simulink model "SIMULINK_FT_SRL_NZS_Tracking_R18b"  (R2018b)
settings: Solver=FixedStepAuto  StartTime=0.0  StopTime=sim_end_time  FixedStep=fixed_step_size  RelTol=1e-3
InitFcn:
  | start_uav_car_10
values from neighbouring files (symbols this model uses):
  a = 1    [start_uav_car_10.m]
  act_end = 2*pi/w1    (= 62.8318530718)    [start_uav_car_10.m]
  b = 1.8    [start_uav_car_10.m]
  battery_threshold = 20    [start_uav_car_10.m]
  bb = 1.2    [start_uav_car_10.m]
  delta_ = [delta_his(2:end,:); delta]    [adp_tracking.m]    (also in start_uav_car_10.m = zeros(N,1))
  draw_gif = false    [start_uav_car_10.m]
  fixed_step_size = 1/30    (= 0.0333333333333)    [start_uav_car_10.m]
  k = 0.2    [start_uav_car_10.m]
  KD_x = 0.000002    (= 2e-06)    [start_uav_car_10.m]
  KD_y = 0.00002    (= 2e-05)    [start_uav_car_10.m]
  kd_z = 0.02    [start_uav_car_10.m]
  KDD_x = 0.0008    [start_uav_car_10.m]
  KDD_y = 0.0008    [start_uav_car_10.m]
  KI_x = 0.000002    (= 2e-06)    [start_uav_car_10.m]
  KI_y = 0.000002    (= 2e-06)    [start_uav_car_10.m]
  ki_z = 0.002    [start_uav_car_10.m]
  KII_x = 0.000000    (= 0)    [start_uav_car_10.m]
  KII_y = 0.000    (= 0)    [start_uav_car_10.m]
  KP_x = 1.5    [start_uav_car_10.m]
  KP_y = 1.5    [start_uav_car_10.m]
  kp_z = 0.7    [start_uav_car_10.m]
  KPP_x = 0.4    [start_uav_car_10.m]
  KPP_y = 0.4    [start_uav_car_10.m]
  lmt = 0.5    [start_uav_car_10.m]
  omega = omega_(i,:)    [adp_tracking.m]    (also in start_uav_car_10.m = 0.3)
  omega_ = [omega_his(2:end,:); omega']    [adp_tracking.m]    (also in start_uav_car_10.m = zeros(N,l))
  R = 200*eye(2)    [adp_tracking.m]    (also in start_uav_car_10.m = 0.7)
  sim_end_time = 300    [start_uav_car_10.m]    (also in trjcar.m = 600)
  UAV_NUM = 1    [start_uav_car_10.m]
  Vel_Switch_1 = 1    [start_uav_car_10.m]
  Vel_Switch_10 = 1    [start_uav_car_10.m]
  Vel_Switch_11 = 1    [start_uav_car_10.m]
  Vel_Switch_12 = 1    [start_uav_car_10.m]
  Vel_Switch_13 = 1    [start_uav_car_10.m]
  Vel_Switch_14 = 1    [start_uav_car_10.m]
  Vel_Switch_15 = 1    [start_uav_car_10.m]
  Vel_Switch_16 = 1    [start_uav_car_10.m]
  Vel_Switch_17 = 1    [start_uav_car_10.m]
  Vel_Switch_18 = 1    [start_uav_car_10.m]
  Vel_Switch_19 = 1    [start_uav_car_10.m]
  Vel_Switch_2 = 1    [start_uav_car_10.m]
  Vel_Switch_20 = 1    [start_uav_car_10.m]
  Vel_Switch_3 = 1    [start_uav_car_10.m]
  Vel_Switch_4 = 1    [start_uav_car_10.m]
  Vel_Switch_5 = 1    [start_uav_car_10.m]
  Vel_Switch_6 = 1    [start_uav_car_10.m]
  Vel_Switch_7 = 1    [start_uav_car_10.m]
  Vel_Switch_8 = 1    [start_uav_car_10.m]
  Vel_Switch_9 = 1    [start_uav_car_10.m]
  W0 = 10*ones(l,1)    [start_uav_car_10.m]
  w1 = 0.1    [start_uav_car_10.m]
  w2 = 30    [start_uav_car_10.m]
  XMAX = 2.8    [start_uav_car_10.m]
  XMIN = -2.8    [start_uav_car_10.m]
  YMAX = 2.2    [start_uav_car_10.m]
  YMIN = -2.2    [start_uav_car_10.m]
  ys = ys_learned - ys_learned(1,:)    [start_uav_car_10.m]
  ys_learned = [-20 -19.9842645881 -19.9722755737 -19.9635643089 -19.9577075469 -19.9543235714 -19.9530686431 -19.9536337356 -19.9557415391 -19.9591437091 -19.9636183405 -19.9689676484 ... (12618 elements, 6309x2)]    [DMP_ref.mat]
  z_d_for_land = 1    [start_uav_car_10.m]
  ZMAX = 2.0    (= 2)    [start_uav_car_10.m]
  ZMIN = 0.7    [start_uav_car_10.m]
undefined symbols (not defined in the file or in its folder): droneyeeUAV2_NUM, droneyeeUAV3_NUM, droneyeeUAV4_NUM, droneyeeUAV5_NUM, uav10num, uav1num, uav2num, uav3num, uav4num, uav5num, uav6num, uav7num, uav8num, uav9num
libraries: simulink x121, aerolibanimutils x1
(part 7 of 11)

== system SIMULINK_FT_SRL_NZS_Tracking_R18b/CMD_UAV/CMD6/Subsystem ==
  clock : Inport
  uavstates : Inport  Port=2
  Constant : Constant  Value=uav6num
  MATLAB Function : MATLAB Function  TreatAsAtomicUnit=on
  "xd " : Outport
  yd : Outport  Port=2
  zd : Outport  Port=3
  wires:
  MATLAB Function/1(x_) -> "xd "/1
  MATLAB Function/2(y_) -> yd/1
  MATLAB Function/3(z_) -> zd/1
  clock/1 -> MATLAB Function/1(timestamp)
  Constant/1 -> MATLAB Function/2(uavnum)
  [switch_flag] -> MATLAB Function/3(switch_flag)
  uavstates/1 -> MATLAB Function/4(stas)
  [trj_flag] -> MATLAB Function/5(trj_flag)
  [form_flag] -> MATLAB Function/6(form_flag)
  [avo_flag] -> MATLAB Function/7(avo_flag)

== system SIMULINK_FT_SRL_NZS_Tracking_R18b/CMD_UAV/CMD7/Subsystem ==
  clock : Inport
  uavstates : Inport  Port=2
  Constant : Constant  Value=uav7num
  MATLAB Function : MATLAB Function  TreatAsAtomicUnit=on
  "xd " : Outport
  yd : Outport  Port=2
  zd : Outport  Port=3
  wires:
  uavstates/1 -> MATLAB Function/4(stas)
  [switch_flag] -> MATLAB Function/3(switch_flag)
  [avo_flag] -> MATLAB Function/7(avo_flag)
  [trj_flag] -> MATLAB Function/5(trj_flag)
  Constant/1 -> MATLAB Function/2(uavnum)
  [form_flag] -> MATLAB Function/6(form_flag)
  clock/1 -> MATLAB Function/1(timestamp)
  MATLAB Function/1(x_) -> "xd "/1
  MATLAB Function/2(y_) -> yd/1
  MATLAB Function/3(z_) -> zd/1

== system SIMULINK_FT_SRL_NZS_Tracking_R18b/CMD_UAV/CMD8/Subsystem ==
  clock : Inport
  uavstates : Inport  Port=2
  Constant : Constant  Value=uav8num
  MATLAB Function : MATLAB Function  TreatAsAtomicUnit=on
  "xd " : Outport
  yd : Outport  Port=2
  zd : Outport  Port=3
  wires:
  MATLAB Function/1(x_) -> "xd "/1
  MATLAB Function/2(y_) -> yd/1
  MATLAB Function/3(z_) -> zd/1
  clock/1 -> MATLAB Function/1(timestamp)
  Constant/1 -> MATLAB Function/2(uavnum)
  [switch_flag] -> MATLAB Function/3(switch_flag)
  uavstates/1 -> MATLAB Function/4(stas)
  [trj_flag] -> MATLAB Function/5(trj_flag)
  [form_flag] -> MATLAB Function/6(form_flag)
  [avo_flag] -> MATLAB Function/7(avo_flag)

== system SIMULINK_FT_SRL_NZS_Tracking_R18b/CMD_UAV/CMD9/Subsystem ==
  clock : Inport
  uavstates : Inport  Port=2
  Constant : Constant  Value=uav9num
  MATLAB Function : MATLAB Function  TreatAsAtomicUnit=on
  "xd " : Outport
  yd : Outport  Port=2
  zd : Outport  Port=3
  wires:
  uavstates/1 -> MATLAB Function/4(stas)
  [switch_flag] -> MATLAB Function/3(switch_flag)
  [avo_flag] -> MATLAB Function/7(avo_flag)
  [trj_flag] -> MATLAB Function/5(trj_flag)
  Constant/1 -> MATLAB Function/2(uavnum)
  [form_flag] -> MATLAB Function/6(form_flag)
  clock/1 -> MATLAB Function/1(timestamp)
  MATLAB Function/1(x_) -> "xd "/1
  MATLAB Function/2(y_) -> yd/1
  MATLAB Function/3(z_) -> zd/1

== system SIMULINK_FT_SRL_NZS_Tracking_R18b/CMD_car1/CMD1/Subsystem ==
  clock : Inport
  uavstates : Inport  Port=2
  Constant : Constant  Value=uav1num
  MATLAB Function : MATLAB Function  TreatAsAtomicUnit=on
  "xd " : Outport
  yd : Outport  Port=2
  zd : Outport  Port=3
  wires:
  MATLAB Function/1(x_) -> "xd "/1
  MATLAB Function/2(y_) -> yd/1
  MATLAB Function/3(z_) -> zd/1
  clock/1 -> MATLAB Function/1(timestamp)
  Constant/1 -> MATLAB Function/2(uavnum)
  [switch_flag] -> MATLAB Function/3(switch_flag)
  uavstates/1 -> MATLAB Function/4(stas)
  [trj_flag] -> MATLAB Function/5(trj_flag)
  [form_flag] -> MATLAB Function/6(form_flag)
  [avo_flag] -> MATLAB Function/7(avo_flag)

== system SIMULINK_FT_SRL_NZS_Tracking_R18b/CMD_car1/CMD10/Subsystem ==
  clock : Inport
  uavstates : Inport  Port=2
  Constant : Constant  Value=uav10num
  Goto : Goto  Commented=on  GotoTag=trj_flag  TagVisibility=global
  Goto1 : Goto  Commented=on  GotoTag=form_flag  TagVisibility=global
  Goto2 : Goto  Commented=on  GotoTag=avo_flag  TagVisibility=global
  MATLAB Function : MATLAB Function  TreatAsAtomicUnit=on
  轨迹 : Constant  Commented=on
  避障 : Constant  Commented=on  Value=0
  队形 : Constant  Commented=on
  "xd " : Outport
  yd : Outport  Port=2
  zd : Outport  Port=3
  wires:
  MATLAB Function/1(x_) -> "xd "/1
  MATLAB Function/2(y_) -> yd/1
  MATLAB Function/3(z_) -> zd/1
  clock/1 -> MATLAB Function/1(timestamp)
  Constant/1 -> MATLAB Function/2(uavnum)
  [switch_flag] -> MATLAB Function/3(switch_flag)
  uavstates/1 -> MATLAB Function/4(stas)
  轨迹/1 -> Goto/1
  队形/1 -> Goto1/1
  避障/1 -> Goto2/1
  [trj_flag] -> MATLAB Function/5(trj_flag)
  [form_flag] -> MATLAB Function/6(form_flag)
  [avo_flag] -> MATLAB Function/7(avo_flag)

== system SIMULINK_FT_SRL_NZS_Tracking_R18b/CMD_car1/CMD2/Subsystem ==
  clock : Inport
  uavstates : Inport  Port=2
  Constant : Constant  Value=uav2num
  MATLAB Function : MATLAB Function  TreatAsAtomicUnit=on
  "xd " : Outport
  yd : Outport  Port=2
  zd : Outport  Port=3
  wires:
  uavstates/1 -> MATLAB Function/4(stas)
  [switch_flag] -> MATLAB Function/3(switch_flag)
  [avo_flag] -> MATLAB Function/7(avo_flag)
  [trj_flag] -> MATLAB Function/5(trj_flag)
  Constant/1 -> MATLAB Function/2(uavnum)
  [form_flag] -> MATLAB Function/6(form_flag)
  clock/1 -> MATLAB Function/1(timestamp)
  MATLAB Function/1(x_) -> "xd "/1
  MATLAB Function/3(z_) -> zd/1
  MATLAB Function/2(y_) -> yd/1

== system SIMULINK_FT_SRL_NZS_Tracking_R18b/CMD_car1/CMD3/Subsystem ==
  clock : Inport
  uavstates : Inport  Port=2
  Constant : Constant  Value=uav3num
  MATLAB Function : MATLAB Function  TreatAsAtomicUnit=on
  "xd " : Outport
  yd : Outport  Port=2
  zd : Outport  Port=3
  wires:
  uavstates/1 -> MATLAB Function/4(stas)
  [switch_flag] -> MATLAB Function/3(switch_flag)
  [avo_flag] -> MATLAB Function/7(avo_flag)
  [trj_flag] -> MATLAB Function/5(trj_flag)
  Constant/1 -> MATLAB Function/2(uavnum)
  [form_flag] -> MATLAB Function/6(form_flag)
  clock/1 -> MATLAB Function/1(timestamp)
  MATLAB Function/1(x_) -> "xd "/1
  MATLAB Function/2(y_) -> yd/1
  MATLAB Function/3(z_) -> zd/1

== system SIMULINK_FT_SRL_NZS_Tracking_R18b/CMD_car1/CMD4/Subsystem ==
  clock : Inport
  uavstates : Inport  Port=2
  Constant : Constant  Value=uav4num
  MATLAB Function : MATLAB Function  TreatAsAtomicUnit=on
  "xd " : Outport
  yd : Outport  Port=2
  zd : Outport  Port=3
  wires:
  uavstates/1 -> MATLAB Function/4(stas)
  [switch_flag] -> MATLAB Function/3(switch_flag)
  [avo_flag] -> MATLAB Function/7(avo_flag)
  [trj_flag] -> MATLAB Function/5(trj_flag)
  Constant/1 -> MATLAB Function/2(uavnum)
  [form_flag] -> MATLAB Function/6(form_flag)
  clock/1 -> MATLAB Function/1(timestamp)
  MATLAB Function/1(x_) -> "xd "/1
  MATLAB Function/2(y_) -> yd/1
  MATLAB Function/3(z_) -> zd/1

== system SIMULINK_FT_SRL_NZS_Tracking_R18b/CMD_car1/CMD5/Subsystem ==
  clock : Inport
  uavstates : Inport  Port=2
  Constant : Constant  Value=uav5num
  MATLAB Function : MATLAB Function  TreatAsAtomicUnit=on
  "xd " : Outport
  yd : Outport  Port=2
  zd : Outport  Port=3
  wires:
  uavstates/1 -> MATLAB Function/4(stas)
  [switch_flag] -> MATLAB Function/3(switch_flag)
  [avo_flag] -> MATLAB Function/7(avo_flag)
  [trj_flag] -> MATLAB Function/5(trj_flag)
  Constant/1 -> MATLAB Function/2(uavnum)
  [form_flag] -> MATLAB Function/6(form_flag)
  clock/1 -> MATLAB Function/1(timestamp)
  MATLAB Function/1(x_) -> "xd "/1
  MATLAB Function/2(y_) -> yd/1
  MATLAB Function/3(z_) -> zd/1

== system SIMULINK_FT_SRL_NZS_Tracking_R18b/CMD_car1/CMD6/Subsystem ==
  clock : Inport
  uavstates : Inport  Port=2
  Constant : Constant  Value=uav6num
  MATLAB Function : MATLAB Function  TreatAsAtomicUnit=on
  "xd " : Outport
  yd : Outport  Port=2
  zd : Outport  Port=3
  wires:
  MATLAB Function/1(x_) -> "xd "/1
  MATLAB Function/2(y_) -> yd/1
  MATLAB Function/3(z_) -> zd/1
  clock/1 -> MATLAB Function/1(timestamp)
  Constant/1 -> MATLAB Function/2(uavnum)
  [switch_flag] -> MATLAB Function/3(switch_flag)
  uavstates/1 -> MATLAB Function/4(stas)
  [trj_flag] -> MATLAB Function/5(trj_flag)
  [form_flag] -> MATLAB Function/6(form_flag)
  [avo_flag] -> MATLAB Function/7(avo_flag)

== system SIMULINK_FT_SRL_NZS_Tracking_R18b/CMD_car1/CMD7/Subsystem ==
  clock : Inport
  uavstates : Inport  Port=2
  Constant : Constant  Value=uav7num
  MATLAB Function : MATLAB Function  TreatAsAtomicUnit=on
  "xd " : Outport
  yd : Outport  Port=2
  zd : Outport  Port=3
  wires:
  uavstates/1 -> MATLAB Function/4(stas)
  [switch_flag] -> MATLAB Function/3(switch_flag)
  [avo_flag] -> MATLAB Function/7(avo_flag)
  [trj_flag] -> MATLAB Function/5(trj_flag)
  Constant/1 -> MATLAB Function/2(uavnum)
  [form_flag] -> MATLAB Function/6(form_flag)
  clock/1 -> MATLAB Function/1(timestamp)
  MATLAB Function/1(x_) -> "xd "/1
  MATLAB Function/2(y_) -> yd/1
  MATLAB Function/3(z_) -> zd/1

== system SIMULINK_FT_SRL_NZS_Tracking_R18b/CMD_car1/CMD8/Subsystem ==
  clock : Inport
  uavstates : Inport  Port=2
  Constant : Constant  Value=uav8num
  MATLAB Function : MATLAB Function  TreatAsAtomicUnit=on
  "xd " : Outport
  yd : Outport  Port=2
  zd : Outport  Port=3
  wires:
  MATLAB Function/1(x_) -> "xd "/1
  MATLAB Function/2(y_) -> yd/1
  MATLAB Function/3(z_) -> zd/1
  clock/1 -> MATLAB Function/1(timestamp)
  Constant/1 -> MATLAB Function/2(uavnum)
  [switch_flag] -> MATLAB Function/3(switch_flag)
  uavstates/1 -> MATLAB Function/4(stas)
  [trj_flag] -> MATLAB Function/5(trj_flag)
  [form_flag] -> MATLAB Function/6(form_flag)
  [avo_flag] -> MATLAB Function/7(avo_flag)

== system SIMULINK_FT_SRL_NZS_Tracking_R18b/CMD_car1/CMD9/Subsystem ==
  clock : Inport
  uavstates : Inport  Port=2
  Constant : Constant  Value=uav9num
  MATLAB Function : MATLAB Function  TreatAsAtomicUnit=on
  "xd " : Outport
  yd : Outport  Port=2
  zd : Outport  Port=3
  wires:
  uavstates/1 -> MATLAB Function/4(stas)
  [switch_flag] -> MATLAB Function/3(switch_flag)
  [avo_flag] -> MATLAB Function/7(avo_flag)
  [trj_flag] -> MATLAB Function/5(trj_flag)
  Constant/1 -> MATLAB Function/2(uavnum)
  [form_flag] -> MATLAB Function/6(form_flag)
  clock/1 -> MATLAB Function/1(timestamp)
  MATLAB Function/1(x_) -> "xd "/1
  MATLAB Function/2(y_) -> yd/1
  MATLAB Function/3(z_) -> zd/1

== system SIMULINK_FT_SRL_NZS_Tracking_R18b/control system_UAV/Baseline Controller1/Heading controller ==
  yaw_e (rad) : Inport
  yaw_d. (rad) : Inport  Port=2
  Integrator Limited : Integrator  Commented=on  LimitOutput=on  UpperSaturationLimit=0.3  LowerSaturationLimit=-0.3
  Ki : Gain  Commented=on  Gain=0.01
  Sum1 : Sum  Inputs=|-+
  Sum2 : Sum  Inputs=|++
  proportional control gain - yaw : Gain  Gain=0.2
  yaw_rate_d. (rad/s) : Outport
  wires:
  Sum1/1 -> Ki/1, proportional control gain - yaw/1
  yaw_e (rad)/1 -> Sum1/1
  yaw_d. (rad)/1 -> Sum1/2
  proportional control gain - yaw/1 -> Sum2/1
  Integrator Limited/1 -> Sum2/2
  Ki/1 -> Integrator Limited/1
  Sum2/1 -> yaw_rate_d. (rad/s)/1

== system SIMULINK_FT_SRL_NZS_Tracking_R18b/control system_UAV/Baseline Controller1/Height controller  ==
  Z_d. (m) : Inport
  Z_e (m) : Inport  Port=2
  V_z : Inport  Port=3
  Discrete Derivative1 : simulink/Discrete/Discrete Derivative  gainval=1.0  ICPrevScaledInput=0.0  OutMin=[]  OutMax=[]  OutDataType=fixdt(1, 16)  OutScaling=2^-10  DoSatur=off
  Integrator Limited : Integrator  LimitOutput=on  UpperSaturationLimit=0.1  LowerSaturationLimit=-0.1
  Kd : Gain  Gain=kd_z
  Ki : Gain  Gain=ki_z
  Kp : Gain  Gain=kp_z
  Sum2 : Sum  Inputs=+++
  Sum3 : Sum  Inputs=|-+
  Z_velocity_d (m/s) : Outport
  wires:
  Sum3/1 -> Discrete Derivative1/1, Ki/1, Kp/1
  Z_e (m)/1 -> Sum3/1
  Discrete Derivative1/1 -> Kd/1
  Sum2/1 -> Z_velocity_d (m/s)/1
  Kp/1 -> Sum2/2
  Kd/1 -> Sum2/3
  Ki/1 -> Integrator Limited/1
  Integrator Limited/1 -> Sum2/1
  Z_d. (m)/1 -> Sum3/2

== system SIMULINK_FT_SRL_NZS_Tracking_R18b/control system_UAV/Baseline Controller1/Position controller ==
  X_e (m) : Inport
  Y_e (m) : Inport  Port=2
  X_d (m) : Inport  Port=3
  Y_d (m) : Inport  Port=4
  Discrete Derivative1 : simulink/Discrete/Discrete Derivative  gainval=1.0  ICPrevScaledInput=0.0  OutMin=[]  OutMax=[]  OutDataType=fixdt(1, 16)  OutScaling=2^-10  DoSatur=off
  Discrete Derivative2 : simulink/Discrete/Discrete Derivative  gainval=1.0  ICPrevScaledInput=0.0  OutMin=[]  OutMax=[]  OutDataType=fixdt(1, 16)  OutScaling=2^-10  DoSatur=off
  Integrator Limited : Integrator  LimitOutput=on  UpperSaturationLimit=0.4  LowerSaturationLimit=-0.4
  Integrator Limited1 : Integrator  LimitOutput=on  UpperSaturationLimit=0.4  LowerSaturationLimit=-0.4
  Kd : Gain  Gain=KD_x
  Kd1 : Gain  Gain=KD_y
  Kp : Gain  Gain=KP_x
  Kp1 : Gain  Gain=KI_x
  Kp2 : Gain  Gain=KP_y
  Kp3 : Gain  Gain=KI_y
  Mux : Mux  Inputs=2
  Sum2 : Sum  Inputs=+++
  Sum3 : Sum  Inputs=|-+
  Sum5 : Sum  Inputs=+++
  Sum6 : Sum  Inputs=|-+
  uxy : Outport
  wires:
  Sum5/1 -> Mux/2
  Discrete Derivative1/1 -> Kd/1
  Kp2/1 -> Sum5/2
  Sum3/1 -> Discrete Derivative1/1, Kp/1, Kp1/1
  Discrete Derivative2/1 -> Kd1/1
  X_d (m)/1 -> Sum3/2
  Integrator Limited/1 -> Sum2/1
  Y_d (m)/1 -> Sum6/2
  Kp3/1 -> Integrator Limited1/1
  Kp1/1 -> Integrator Limited/1
  Kd1/1 -> Sum5/3
  Mux/1 -> uxy/1
  Kp/1 -> Sum2/2
  X_e (m)/1 -> Sum3/1
  Integrator Limited1/1 -> Sum5/1
  Sum2/1 -> Mux/1
  Kd/1 -> Sum2/3
  Y_e (m)/1 -> Sum6/1
  Sum6/1 -> Discrete Derivative2/1, Kp2/1, Kp3/1

== system SIMULINK_FT_SRL_NZS_Tracking_R18b/control system_UAV/Baseline Controller10/Heading controller ==
  yaw_e (rad) : Inport
  yaw_d. (rad) : Inport  Port=2
  Integrator Limited : Integrator  Commented=on  LimitOutput=on  UpperSaturationLimit=0.3  LowerSaturationLimit=-0.3
  Ki : Gain  Commented=on  Gain=0.01
  Sum1 : Sum  Inputs=|-+
  Sum2 : Sum  Inputs=|++
  proportional control gain - yaw : Gain  Gain=0.2
  yaw_rate_d. (rad/s) : Outport
  wires:
  Sum1/1 -> Ki/1, proportional control gain - yaw/1
  yaw_e (rad)/1 -> Sum1/1
  yaw_d. (rad)/1 -> Sum1/2
  proportional control gain - yaw/1 -> Sum2/1
  Integrator Limited/1 -> Sum2/2
  Ki/1 -> Integrator Limited/1
  Sum2/1 -> yaw_rate_d. (rad/s)/1

== system SIMULINK_FT_SRL_NZS_Tracking_R18b/control system_UAV/Baseline Controller10/Height controller  ==
  Z_d. (m) : Inport
  Z_e (m) : Inport  Port=2
  V_z : Inport  Port=3
  Discrete Derivative1 : simulink/Discrete/Discrete Derivative  gainval=1.0  ICPrevScaledInput=0.0  OutMin=[]  OutMax=[]  OutDataType=fixdt(1, 16)  OutScaling=2^-10  DoSatur=off
  Integrator Limited : Integrator  LimitOutput=on  UpperSaturationLimit=0.1  LowerSaturationLimit=-0.1
  Kd : Gain  Gain=kd_z
  Ki : Gain  Gain=ki_z
  Kp : Gain  Gain=kp_z
  Sum2 : Sum  Inputs=+++
  Sum3 : Sum  Inputs=|-+
  Z_velocity_d (m/s) : Outport
  wires:
  Sum3/1 -> Discrete Derivative1/1, Ki/1, Kp/1
  Z_e (m)/1 -> Sum3/1
  Discrete Derivative1/1 -> Kd/1
  Sum2/1 -> Z_velocity_d (m/s)/1
  Kp/1 -> Sum2/2
  Kd/1 -> Sum2/3
  Ki/1 -> Integrator Limited/1
  Integrator Limited/1 -> Sum2/1
  Z_d. (m)/1 -> Sum3/2

== system SIMULINK_FT_SRL_NZS_Tracking_R18b/control system_UAV/Baseline Controller10/Position controller ==
  X_e (m) : Inport
  Y_e (m) : Inport  Port=2
  X_d (m) : Inport  Port=3
  Y_d (m) : Inport  Port=4
  Discrete Derivative1 : simulink/Discrete/Discrete Derivative  gainval=1.0  ICPrevScaledInput=0.0  OutMin=[]  OutMax=[]  OutDataType=fixdt(1, 16)  OutScaling=2^-10  DoSatur=off
  Discrete Derivative2 : simulink/Discrete/Discrete Derivative  gainval=1.0  ICPrevScaledInput=0.0  OutMin=[]  OutMax=[]  OutDataType=fixdt(1, 16)  OutScaling=2^-10  DoSatur=off
  Integrator Limited : Integrator  LimitOutput=on  UpperSaturationLimit=0.5  LowerSaturationLimit=-0.5
  Integrator Limited1 : Integrator  LimitOutput=on  UpperSaturationLimit=0.5  LowerSaturationLimit=-0.5
  Kd : Gain  Gain=KD_x
  Kd1 : Gain  Gain=KD_y
  Kp : Gain  Gain=KP_x
  Kp1 : Gain  Gain=KI_x
  Kp2 : Gain  Gain=KP_y
  Kp3 : Gain  Gain=KI_y
  Mux : Mux  Inputs=2
  Scope : Scope
  Scope1 : Scope
  Sum2 : Sum  Inputs=+++
  Sum3 : Sum  Inputs=|-+
  Sum5 : Sum  Inputs=+++
  Sum6 : Sum  Inputs=|-+
  uxy : Outport
  wires:
  X_e (m)/1 -> Sum3/1
  Integrator Limited/1 -> Sum2/1
  Sum2/1 -> Mux/1, Scope/1
  Kp1/1 -> Integrator Limited/1
  Kp/1 -> Sum2/2
  Kp2/1 -> Sum5/2
  Y_e (m)/1 -> Sum6/1
  Integrator Limited1/1 -> Sum5/1
  Sum5/1 -> Mux/2, Scope1/1
  Kp3/1 -> Integrator Limited1/1
  Mux/1 -> uxy/1
  X_d (m)/1 -> Sum3/2
  Discrete Derivative1/1 -> Kd/1
  Sum3/1 -> Discrete Derivative1/1, Kp/1, Kp1/1
  Y_d (m)/1 -> Sum6/2
  Sum6/1 -> Discrete Derivative2/1, Kp2/1, Kp3/1
  Kd1/1 -> Sum5/3
  Discrete Derivative2/1 -> Kd1/1
  Kd/1 -> Sum2/3

== system SIMULINK_FT_SRL_NZS_Tracking_R18b/control system_UAV/Baseline Controller2/Heading controller ==
  yaw_e (rad) : Inport
  yaw_d. (rad) : Inport  Port=2
  Integrator Limited : Integrator  Commented=on  LimitOutput=on  UpperSaturationLimit=0.3  LowerSaturationLimit=-0.3
  Ki : Gain  Commented=on  Gain=0.01
  Sum1 : Sum  Inputs=|-+
  Sum2 : Sum  Inputs=|++
  proportional control gain - yaw : Gain  Gain=0.2
  yaw_rate_d. (rad/s) : Outport
  wires:
  Sum2/1 -> yaw_rate_d. (rad/s)/1
  Ki/1 -> Integrator Limited/1
  Integrator Limited/1 -> Sum2/2
  proportional control gain - yaw/1 -> Sum2/1
  yaw_d. (rad)/1 -> Sum1/2
  yaw_e (rad)/1 -> Sum1/1
  Sum1/1 -> proportional control gain - yaw/1, Ki/1

== system SIMULINK_FT_SRL_NZS_Tracking_R18b/control system_UAV/Baseline Controller2/Height controller  ==
  Z_d. (m) : Inport
  Z_e (m) : Inport  Port=2
  V_z : Inport  Port=3
  Discrete Derivative1 : simulink/Discrete/Discrete Derivative  gainval=1.0  ICPrevScaledInput=0.0  OutMin=[]  OutMax=[]  OutDataType=fixdt(1, 16)  OutScaling=2^-10  DoSatur=off
  Integrator Limited : Integrator  LimitOutput=on  UpperSaturationLimit=0.1  LowerSaturationLimit=-0.1
  Kd : Gain  Gain=kd_z
  Ki : Gain  Gain=ki_z
  Kp : Gain  Gain=kp_z
  Sum2 : Sum  Inputs=+++
  Sum3 : Sum  Inputs=|-+
  Z_velocity_d (m/s) : Outport
  wires:
  Sum3/1 -> Discrete Derivative1/1, Ki/1, Kp/1
  Z_e (m)/1 -> Sum3/1
  Discrete Derivative1/1 -> Kd/1
  Sum2/1 -> Z_velocity_d (m/s)/1
  Kp/1 -> Sum2/2
  Kd/1 -> Sum2/3
  Ki/1 -> Integrator Limited/1
  Integrator Limited/1 -> Sum2/1
  Z_d. (m)/1 -> Sum3/2

== system SIMULINK_FT_SRL_NZS_Tracking_R18b/control system_UAV/Baseline Controller2/Position controller ==
  X_e (m) : Inport
  Y_e (m) : Inport  Port=2
  X_d (m) : Inport  Port=3
  Y_d (m) : Inport  Port=4
  Discrete Derivative1 : simulink/Discrete/Discrete Derivative  gainval=1.0  ICPrevScaledInput=0.0  OutMin=[]  OutMax=[]  OutDataType=fixdt(1, 16)  OutScaling=2^-10  DoSatur=off
  Discrete Derivative2 : simulink/Discrete/Discrete Derivative  gainval=1.0  ICPrevScaledInput=0.0  OutMin=[]  OutMax=[]  OutDataType=fixdt(1, 16)  OutScaling=2^-10  DoSatur=off
  Integrator Limited : Integrator  LimitOutput=on  UpperSaturationLimit=0.4  LowerSaturationLimit=-0.4
  Integrator Limited1 : Integrator  LimitOutput=on  UpperSaturationLimit=0.4  LowerSaturationLimit=-0.4
  Kd : Gain  Gain=KD_x
  Kd1 : Gain  Gain=KD_y
  Kp : Gain  Gain=KP_x
  Kp1 : Gain  Gain=KI_x
  Kp2 : Gain  Gain=KP_y
  Kp3 : Gain  Gain=KI_y
  Mux : Mux  Inputs=2
  Sum2 : Sum  Inputs=+++
  Sum3 : Sum  Inputs=|-+
  Sum5 : Sum  Inputs=+++
  Sum6 : Sum  Inputs=|-+
  uxy : Outport
  wires:
  Discrete Derivative2/1 -> Kd1/1
  Kd1/1 -> Sum5/3
  Sum6/1 -> Discrete Derivative2/1, Kp2/1, Kp3/1
  Y_d (m)/1 -> Sum6/2
  Kd/1 -> Sum2/3
  Discrete Derivative1/1 -> Kd/1
  Sum3/1 -> Discrete Derivative1/1, Kp1/1, Kp/1
  X_d (m)/1 -> Sum3/2
  Mux/1 -> uxy/1
  Kp3/1 -> Integrator Limited1/1
  Integrator Limited1/1 -> Sum5/1
  Y_e (m)/1 -> Sum6/1
  Kp2/1 -> Sum5/2
  Kp/1 -> Sum2/2
  Kp1/1 -> Integrator Limited/1
  Integrator Limited/1 -> Sum2/1
  X_e (m)/1 -> Sum3/1
  Sum2/1 -> Mux/1
  Sum5/1 -> Mux/2

== system SIMULINK_FT_SRL_NZS_Tracking_R18b/control system_UAV/Baseline Controller3/Heading controller ==
  yaw_e (rad) : Inport
  yaw_d. (rad) : Inport  Port=2
  Integrator Limited : Integrator  Commented=on  LimitOutput=on  UpperSaturationLimit=0.3  LowerSaturationLimit=-0.3
  Ki : Gain  Commented=on  Gain=0.01
  Sum1 : Sum  Inputs=|-+
  Sum2 : Sum  Inputs=|++
  proportional control gain - yaw : Gain  Gain=0.2
  yaw_rate_d. (rad/s) : Outport
  wires:
  Sum1/1 -> Ki/1, proportional control gain - yaw/1
  yaw_e (rad)/1 -> Sum1/1
  yaw_d. (rad)/1 -> Sum1/2
  proportional control gain - yaw/1 -> Sum2/1
  Integrator Limited/1 -> Sum2/2
  Ki/1 -> Integrator Limited/1
  Sum2/1 -> yaw_rate_d. (rad/s)/1

== system SIMULINK_FT_SRL_NZS_Tracking_R18b/control system_UAV/Baseline Controller3/Height controller  ==
  Z_d. (m) : Inport
  Z_e (m) : Inport  Port=2
  V_z : Inport  Port=3
  Discrete Derivative1 : simulink/Discrete/Discrete Derivative  gainval=1.0  ICPrevScaledInput=0.0  OutMin=[]  OutMax=[]  OutDataType=fixdt(1, 16)  OutScaling=2^-10  DoSatur=off
  Integrator Limited : Integrator  LimitOutput=on  UpperSaturationLimit=0.1  LowerSaturationLimit=-0.1
  Kd : Gain  Gain=kd_z
  Ki : Gain  Gain=ki_z
  Kp : Gain  Gain=kp_z
  Sum2 : Sum  Inputs=+++
  Sum3 : Sum  Inputs=|-+
  Z_velocity_d (m/s) : Outport
  wires:
  Sum3/1 -> Discrete Derivative1/1, Ki/1, Kp/1
  Z_e (m)/1 -> Sum3/1
  Discrete Derivative1/1 -> Kd/1
  Sum2/1 -> Z_velocity_d (m/s)/1
  Kp/1 -> Sum2/2
  Kd/1 -> Sum2/3
  Ki/1 -> Integrator Limited/1
  Integrator Limited/1 -> Sum2/1
  Z_d. (m)/1 -> Sum3/2

== system SIMULINK_FT_SRL_NZS_Tracking_R18b/control system_UAV/Baseline Controller3/Position controller ==
  X_e (m) : Inport
  Y_e (m) : Inport  Port=2
  X_d (m) : Inport  Port=3
  Y_d (m) : Inport  Port=4
  Constant : Constant  Value=0
  Discrete Derivative1 : simulink/Discrete/Discrete Derivative  gainval=1.0  ICPrevScaledInput=0.0  OutMin=[]  OutMax=[]  OutDataType=fixdt(1, 16)  OutScaling=2^-10  DoSatur=off
  Discrete Derivative2 : simulink/Discrete/Discrete Derivative  gainval=1.0  ICPrevScaledInput=0.0  OutMin=[]  OutMax=[]  OutDataType=fixdt(1, 16)  OutScaling=2^-10  DoSatur=off
  Integrator Limited : Integrator  LimitOutput=on  UpperSaturationLimit=0.5  LowerSaturationLimit=-0.5
  Integrator Limited1 : Integrator  LimitOutput=on  UpperSaturationLimit=0.5  LowerSaturationLimit=-0.5
  Kd : Gain  Gain=KD_x
  Kd1 : Gain  Gain=KD_y
  Kp : Gain  Gain=KP_x
  Kp1 : Gain  Gain=KI_x
  Kp2 : Gain  Gain=KP_y
  Kp3 : Gain  Gain=KI_y
  MATLAB Function : MATLAB Function  TreatAsAtomicUnit=on
  MATLAB Function1 : MATLAB Function  TreatAsAtomicUnit=on
  Mux : Mux  Inputs=2
  Mux1 : Mux  Inputs=2
  Mux2 : Mux  Inputs=2
  Scope1 : Scope  NumInputPorts=2
  Sum2 : Sum  Inputs=+++
  Sum3 : Sum  Inputs=|-+
  Sum5 : Sum  Inputs=+++
  Sum6 : Sum  Inputs=|-+
  Terminator : Terminator
  Terminator1 : Terminator
  To Workspace : ToWorkspace  VariableName=u  SaveFormat=Timeseries  SampleTime=-1
  To Workspace1 : ToWorkspace  VariableName=u2  SaveFormat=Timeseries  SampleTime=-1
  X-Y ADP tracking controller : Subsystem
  position_x_xd : Scope  NumInputPorts=2
  uxy : Outport
  u2xy : Outport  Port=2
  wires:
  Integrator Limited/1 -> Sum2/1
  Kp1/1 -> Integrator Limited/1
  Kp/1 -> Sum2/2
  Kp2/1 -> Sum5/2
  Integrator Limited1/1 -> Sum5/1
  Kp3/1 -> Integrator Limited1/1
  Mux/1 -> Terminator1/1
  Discrete Derivative1/1 -> Kd/1
  Kd/1 -> Sum2/3
  Sum3/1 -> Discrete Derivative1/1, Kp/1, Kp1/1
  Sum6/1 -> Discrete Derivative2/1, Kp2/1, Kp3/1
  Kd1/1 -> Sum5/3
  Discrete Derivative2/1 -> Kd1/1
  Sum2/1 -> Mux/1
  Sum5/1 -> Mux/2
  X-Y ADP tracking controller/2(uy) -> Scope1/2, Mux1/2
  X_d (m)/1 -> MATLAB Function/1(x), Sum3/2
  MATLAB Function1/1(p) -> position_x_xd/1, X-Y ADP tracking controller/1(Feedback1)
  Y_d (m)/1 -> MATLAB Function/2(y), Sum6/2
  X_e (m)/1 -> MATLAB Function1/1(x), Sum3/1
  Mux1/1 -> To Workspace/1, uxy/1
  X-Y ADP tracking controller/3(" p_virtual1") -> Terminator/1
  Y_e (m)/1 -> MATLAB Function1/2(y), Sum6/1
  MATLAB Function/1(p) -> position_x_xd/2, X-Y ADP tracking controller/3(p_virtual)
  X-Y ADP tracking controller/1(ux) -> Mux1/1, Scope1/1
  Constant/1 -> X-Y ADP tracking controller/2(Joystick)
  Mux2/1 -> u2xy/1, To Workspace1/1
  X-Y ADP tracking controller/4(u2x) -> Mux2/1
  X-Y ADP tracking controller/5(u2y) -> Mux2/2

== system SIMULINK_FT_SRL_NZS_Tracking_R18b/control system_UAV/Baseline Controller4/Heading controller ==
  yaw_e (rad) : Inport
  yaw_d. (rad) : Inport  Port=2
  Integrator Limited : Integrator  Commented=on  LimitOutput=on  UpperSaturationLimit=0.3  LowerSaturationLimit=-0.3
  Ki : Gain  Commented=on  Gain=0.01
  Sum1 : Sum  Inputs=|-+
  Sum2 : Sum  Inputs=|++
  proportional control gain - yaw : Gain  Gain=0.2
  yaw_rate_d. (rad/s) : Outport
  wires:
  Sum2/1 -> yaw_rate_d. (rad/s)/1
  Ki/1 -> Integrator Limited/1
  Integrator Limited/1 -> Sum2/2
  proportional control gain - yaw/1 -> Sum2/1
  yaw_d. (rad)/1 -> Sum1/2
  yaw_e (rad)/1 -> Sum1/1
  Sum1/1 -> proportional control gain - yaw/1, Ki/1

== system SIMULINK_FT_SRL_NZS_Tracking_R18b/control system_UAV/Baseline Controller4/Height controller  ==
  Z_d. (m) : Inport
  Z_e (m) : Inport  Port=2
  V_z : Inport  Port=3
  Discrete Derivative1 : simulink/Discrete/Discrete Derivative  gainval=1.0  ICPrevScaledInput=0.0  OutMin=[]  OutMax=[]  OutDataType=fixdt(1, 16)  OutScaling=2^-10  DoSatur=off
  Integrator Limited : Integrator  LimitOutput=on  UpperSaturationLimit=0.1  LowerSaturationLimit=-0.1
  Kd : Gain  Gain=kd_z
  Ki : Gain  Gain=ki_z
  Kp : Gain  Gain=kp_z
  Sum2 : Sum  Inputs=+++
  Sum3 : Sum  Inputs=|-+
  Z_velocity_d (m/s) : Outport
  wires:
  Sum3/1 -> Discrete Derivative1/1, Ki/1, Kp/1
  Z_e (m)/1 -> Sum3/1
  Discrete Derivative1/1 -> Kd/1
  Sum2/1 -> Z_velocity_d (m/s)/1
  Kp/1 -> Sum2/2
  Kd/1 -> Sum2/3
  Ki/1 -> Integrator Limited/1
  Integrator Limited/1 -> Sum2/1
  Z_d. (m)/1 -> Sum3/2

== system SIMULINK_FT_SRL_NZS_Tracking_R18b/control system_UAV/Baseline Controller4/Position controller ==
  X_e (m) : Inport
  Y_e (m) : Inport  Port=2
  X_d (m) : Inport  Port=3
  Y_d (m) : Inport  Port=4
  Discrete Derivative1 : simulink/Discrete/Discrete Derivative  gainval=1.0  ICPrevScaledInput=0.0  OutMin=[]  OutMax=[]  OutDataType=fixdt(1, 16)  OutScaling=2^-10  DoSatur=off
  Discrete Derivative2 : simulink/Discrete/Discrete Derivative  gainval=1.0  ICPrevScaledInput=0.0  OutMin=[]  OutMax=[]  OutDataType=fixdt(1, 16)  OutScaling=2^-10  DoSatur=off
  Integrator Limited : Integrator  LimitOutput=on  UpperSaturationLimit=0.5  LowerSaturationLimit=-0.5
  Integrator Limited1 : Integrator  LimitOutput=on  UpperSaturationLimit=0.5  LowerSaturationLimit=-0.5
  Kd : Gain  Gain=KD_x
  Kd1 : Gain  Gain=KD_y
  Kp : Gain  Gain=KP_x
  Kp1 : Gain  Gain=KI_x
  Kp2 : Gain  Gain=KP_y
  Kp3 : Gain  Gain=KI_y
  Mux : Mux  Inputs=2
  Sum2 : Sum  Inputs=+++
  Sum3 : Sum  Inputs=|-+
  Sum5 : Sum  Inputs=+++
  Sum6 : Sum  Inputs=|-+
  uxy : Outport
  wires:
  Discrete Derivative2/1 -> Kd1/1
  Kd1/1 -> Sum5/3
  Sum6/1 -> Discrete Derivative2/1, Kp3/1, Kp2/1
  Y_d (m)/1 -> Sum6/2
  Sum3/1 -> Discrete Derivative1/1, Kp1/1, Kp/1
  Kd/1 -> Sum2/3
  Discrete Derivative1/1 -> Kd/1
  X_d (m)/1 -> Sum3/2
  Mux/1 -> uxy/1
  Kp3/1 -> Integrator Limited1/1
  Integrator Limited1/1 -> Sum5/1
  Y_e (m)/1 -> Sum6/1
  Kp2/1 -> Sum5/2
  Kp/1 -> Sum2/2
  Kp1/1 -> Integrator Limited/1
  Integrator Limited/1 -> Sum2/1
  X_e (m)/1 -> Sum3/1
  Sum5/1 -> Mux/2
  Sum2/1 -> Mux/1

== system SIMULINK_FT_SRL_NZS_Tracking_R18b/control system_UAV/Baseline Controller5/Heading controller ==
  yaw_e (rad) : Inport
  yaw_d. (rad) : Inport  Port=2
  Integrator Limited : Integrator  Commented=on  LimitOutput=on  UpperSaturationLimit=0.3  LowerSaturationLimit=-0.3
  Ki : Gain  Commented=on  Gain=0.01
  Sum1 : Sum  Inputs=|-+
  Sum2 : Sum  Inputs=|++
  proportional control gain - yaw : Gain  Gain=0.2
  yaw_rate_d. (rad/s) : Outport
  wires:
  Sum1/1 -> Ki/1, proportional control gain - yaw/1
  yaw_e (rad)/1 -> Sum1/1
  yaw_d. (rad)/1 -> Sum1/2
  proportional control gain - yaw/1 -> Sum2/1
  Integrator Limited/1 -> Sum2/2
  Ki/1 -> Integrator Limited/1
  Sum2/1 -> yaw_rate_d. (rad/s)/1

== system SIMULINK_FT_SRL_NZS_Tracking_R18b/control system_UAV/Baseline Controller5/Height controller  ==
  Z_d. (m) : Inport
  Z_e (m) : Inport  Port=2
  V_z : Inport  Port=3
  Discrete Derivative1 : simulink/Discrete/Discrete Derivative  gainval=1.0  ICPrevScaledInput=0.0  OutMin=[]  OutMax=[]  OutDataType=fixdt(1, 16)  OutScaling=2^-10  DoSatur=off
  Integrator Limited : Integrator  LimitOutput=on  UpperSaturationLimit=0.1  LowerSaturationLimit=-0.1
  Kd : Gain  Gain=kd_z
  Ki : Gain  Gain=ki_z
  Kp : Gain  Gain=kp_z
  Sum2 : Sum  Inputs=+++
  Sum3 : Sum  Inputs=|-+
  Z_velocity_d (m/s) : Outport
  wires:
  Sum3/1 -> Discrete Derivative1/1, Ki/1, Kp/1
  Z_e (m)/1 -> Sum3/1
  Discrete Derivative1/1 -> Kd/1
  Sum2/1 -> Z_velocity_d (m/s)/1
  Kp/1 -> Sum2/2
  Kd/1 -> Sum2/3
  Ki/1 -> Integrator Limited/1
  Integrator Limited/1 -> Sum2/1
  Z_d. (m)/1 -> Sum3/2

== system SIMULINK_FT_SRL_NZS_Tracking_R18b/control system_UAV/Baseline Controller5/Position controller ==
  X_e (m) : Inport
  Y_e (m) : Inport  Port=2
  X_d (m) : Inport  Port=3
  Y_d (m) : Inport  Port=4
  Discrete Derivative1 : simulink/Discrete/Discrete Derivative  gainval=1.0  ICPrevScaledInput=0.0  OutMin=[]  OutMax=[]  OutDataType=fixdt(1, 16)  OutScaling=2^-10  DoSatur=off
  Discrete Derivative2 : simulink/Discrete/Discrete Derivative  gainval=1.0  ICPrevScaledInput=0.0  OutMin=[]  OutMax=[]  OutDataType=fixdt(1, 16)  OutScaling=2^-10  DoSatur=off
  Integrator Limited : Integrator  LimitOutput=on  UpperSaturationLimit=0.5  LowerSaturationLimit=-0.5
  Integrator Limited1 : Integrator  LimitOutput=on  UpperSaturationLimit=0.5  LowerSaturationLimit=-0.5
  Kd : Gain  Gain=KD_x
  Kd1 : Gain  Gain=KD_y
  Kp : Gain  Gain=KP_x
  Kp1 : Gain  Gain=KI_x
  Kp2 : Gain  Gain=KP_y
  Kp3 : Gain  Gain=KI_y
  Mux : Mux  Inputs=2
  Scope : Scope
  Scope1 : Scope
  Sum2 : Sum  Inputs=+++
  Sum3 : Sum  Inputs=|-+
  Sum5 : Sum  Inputs=+++
  Sum6 : Sum  Inputs=|-+
  uxy : Outport
  wires:
  X_e (m)/1 -> Sum3/1
  Integrator Limited/1 -> Sum2/1
  Sum2/1 -> Mux/1, Scope/1
  Kp1/1 -> Integrator Limited/1
  Kp/1 -> Sum2/2
  Kp2/1 -> Sum5/2
  Y_e (m)/1 -> Sum6/1
  Integrator Limited1/1 -> Sum5/1
  Sum5/1 -> Mux/2, Scope1/1
  Kp3/1 -> Integrator Limited1/1
  Mux/1 -> uxy/1
  X_d (m)/1 -> Sum3/2
  Discrete Derivative1/1 -> Kd/1
  Sum3/1 -> Discrete Derivative1/1, Kp/1, Kp1/1
  Y_d (m)/1 -> Sum6/2
  Sum6/1 -> Discrete Derivative2/1, Kp2/1, Kp3/1
  Kd1/1 -> Sum5/3
  Discrete Derivative2/1 -> Kd1/1
  Kd/1 -> Sum2/3

== system SIMULINK_FT_SRL_NZS_Tracking_R18b/control system_UAV/Baseline Controller6/Heading controller ==
  yaw_e (rad) : Inport
  yaw_d. (rad) : Inport  Port=2
  Integrator Limited : Integrator  Commented=on  LimitOutput=on  UpperSaturationLimit=0.3  LowerSaturationLimit=-0.3
  Ki : Gain  Commented=on  Gain=0.01
  Sum1 : Sum  Inputs=|-+
  Sum2 : Sum  Inputs=|++
  proportional control gain - yaw : Gain  Gain=0.2
  yaw_rate_d. (rad/s) : Outport
  wires:
  Sum1/1 -> Ki/1, proportional control gain - yaw/1
  yaw_e (rad)/1 -> Sum1/1
  yaw_d. (rad)/1 -> Sum1/2
  proportional control gain - yaw/1 -> Sum2/1
  Integrator Limited/1 -> Sum2/2
  Ki/1 -> Integrator Limited/1
  Sum2/1 -> yaw_rate_d. (rad/s)/1

== system SIMULINK_FT_SRL_NZS_Tracking_R18b/control system_UAV/Baseline Controller6/Height controller  ==
  Z_d. (m) : Inport
  Z_e (m) : Inport  Port=2
  V_z : Inport  Port=3
  Discrete Derivative1 : simulink/Discrete/Discrete Derivative  gainval=1.0  ICPrevScaledInput=0.0  OutMin=[]  OutMax=[]  OutDataType=fixdt(1, 16)  OutScaling=2^-10  DoSatur=off
  Integrator Limited : Integrator  LimitOutput=on  UpperSaturationLimit=0.1  LowerSaturationLimit=-0.1
  Kd : Gain  Gain=kd_z
  Ki : Gain  Gain=ki_z
  Kp : Gain  Gain=kp_z
  Sum2 : Sum  Inputs=+++
  Sum3 : Sum  Inputs=|-+
  Z_velocity_d (m/s) : Outport
  wires:
  Sum3/1 -> Discrete Derivative1/1, Ki/1, Kp/1
  Z_e (m)/1 -> Sum3/1
  Discrete Derivative1/1 -> Kd/1
  Sum2/1 -> Z_velocity_d (m/s)/1
  Kp/1 -> Sum2/2
  Kd/1 -> Sum2/3
  Ki/1 -> Integrator Limited/1
  Integrator Limited/1 -> Sum2/1
  Z_d. (m)/1 -> Sum3/2

== system SIMULINK_FT_SRL_NZS_Tracking_R18b/control system_UAV/Baseline Controller6/Position controller ==
  X_e (m) : Inport
  Y_e (m) : Inport  Port=2
  X_d (m) : Inport  Port=3
  Y_d (m) : Inport  Port=4
  Discrete Derivative1 : simulink/Discrete/Discrete Derivative  gainval=1.0  ICPrevScaledInput=0.0  OutMin=[]  OutMax=[]  OutDataType=fixdt(1, 16)  OutScaling=2^-10  DoSatur=off
  Discrete Derivative2 : simulink/Discrete/Discrete Derivative  gainval=1.0  ICPrevScaledInput=0.0  OutMin=[]  OutMax=[]  OutDataType=fixdt(1, 16)  OutScaling=2^-10  DoSatur=off
  Integrator Limited : Integrator  LimitOutput=on  UpperSaturationLimit=0.5  LowerSaturationLimit=-0.5
  Integrator Limited1 : Integrator  LimitOutput=on  UpperSaturationLimit=0.5  LowerSaturationLimit=-0.5
  Kd : Gain  Gain=KD_x
  Kd1 : Gain  Gain=KD_y
  Kp : Gain  Gain=KP_x
  Kp1 : Gain  Gain=KI_x
  Kp2 : Gain  Gain=KP_y
  Kp3 : Gain  Gain=KI_y
  Mux : Mux  Inputs=2
  Scope : Scope
  Scope1 : Scope
  Sum2 : Sum  Inputs=+++
  Sum3 : Sum  Inputs=|-+
  Sum5 : Sum  Inputs=+++
  Sum6 : Sum  Inputs=|-+
  uxy : Outport
  wires:
  X_e (m)/1 -> Sum3/1
  Integrator Limited/1 -> Sum2/1
  Sum2/1 -> Mux/1, Scope/1
  Kp1/1 -> Integrator Limited/1
  Kp/1 -> Sum2/2
  Kp2/1 -> Sum5/2
  Y_e (m)/1 -> Sum6/1
  Integrator Limited1/1 -> Sum5/1
  Sum5/1 -> Mux/2, Scope1/1
  Kp3/1 -> Integrator Limited1/1
  Mux/1 -> uxy/1
  X_d (m)/1 -> Sum3/2
  Discrete Derivative1/1 -> Kd/1
  Sum3/1 -> Discrete Derivative1/1, Kp/1, Kp1/1
  Y_d (m)/1 -> Sum6/2
  Sum6/1 -> Discrete Derivative2/1, Kp2/1, Kp3/1
  Kd1/1 -> Sum5/3
  Discrete Derivative2/1 -> Kd1/1
  Kd/1 -> Sum2/3

== system SIMULINK_FT_SRL_NZS_Tracking_R18b/control system_UAV/Baseline Controller7/Heading controller ==
  yaw_e (rad) : Inport
  yaw_d. (rad) : Inport  Port=2
  Integrator Limited : Integrator  Commented=on  LimitOutput=on  UpperSaturationLimit=0.3  LowerSaturationLimit=-0.3
  Ki : Gain  Commented=on  Gain=0.01
  Sum1 : Sum  Inputs=|-+
  Sum2 : Sum  Inputs=|++
  proportional control gain - yaw : Gain  Gain=0.2
  yaw_rate_d. (rad/s) : Outport
  wires:
  Sum1/1 -> Ki/1, proportional control gain - yaw/1
  yaw_e (rad)/1 -> Sum1/1
  yaw_d. (rad)/1 -> Sum1/2
  proportional control gain - yaw/1 -> Sum2/1
  Integrator Limited/1 -> Sum2/2
  Ki/1 -> Integrator Limited/1
  Sum2/1 -> yaw_rate_d. (rad/s)/1

== system SIMULINK_FT_SRL_NZS_Tracking_R18b/control system_UAV/Baseline Controller7/Height controller  ==
  Z_d. (m) : Inport
  Z_e (m) : Inport  Port=2
  V_z : Inport  Port=3
  Discrete Derivative1 : simulink/Discrete/Discrete Derivative  gainval=1.0  ICPrevScaledInput=0.0  OutMin=[]  OutMax=[]  OutDataType=fixdt(1, 16)  OutScaling=2^-10  DoSatur=off
  Integrator Limited : Integrator  LimitOutput=on  UpperSaturationLimit=0.1  LowerSaturationLimit=-0.1
  Kd : Gain  Gain=kd_z
  Ki : Gain  Gain=ki_z
  Kp : Gain  Gain=kp_z
  Sum2 : Sum  Inputs=+++
  Sum3 : Sum  Inputs=|-+
  Z_velocity_d (m/s) : Outport
  wires:
  Sum3/1 -> Discrete Derivative1/1, Ki/1, Kp/1
  Z_e (m)/1 -> Sum3/1
  Discrete Derivative1/1 -> Kd/1
  Sum2/1 -> Z_velocity_d (m/s)/1
  Kp/1 -> Sum2/2
  Kd/1 -> Sum2/3
  Ki/1 -> Integrator Limited/1
  Integrator Limited/1 -> Sum2/1
  Z_d. (m)/1 -> Sum3/2

== system SIMULINK_FT_SRL_NZS_Tracking_R18b/control system_UAV/Baseline Controller7/Position controller ==
  X_e (m) : Inport
  Y_e (m) : Inport  Port=2
  X_d (m) : Inport  Port=3
  Y_d (m) : Inport  Port=4
  Discrete Derivative1 : simulink/Discrete/Discrete Derivative  gainval=1.0  ICPrevScaledInput=0.0  OutMin=[]  OutMax=[]  OutDataType=fixdt(1, 16)  OutScaling=2^-10  DoSatur=off
  Discrete Derivative2 : simulink/Discrete/Discrete Derivative  gainval=1.0  ICPrevScaledInput=0.0  OutMin=[]  OutMax=[]  OutDataType=fixdt(1, 16)  OutScaling=2^-10  DoSatur=off
  Integrator Limited : Integrator  LimitOutput=on  UpperSaturationLimit=0.5  LowerSaturationLimit=-0.5
  Integrator Limited1 : Integrator  LimitOutput=on  UpperSaturationLimit=0.5  LowerSaturationLimit=-0.5
  Kd : Gain  Gain=KD_x
  Kd1 : Gain  Gain=KD_y
  Kp : Gain  Gain=KP_x
  Kp1 : Gain  Gain=KI_x
  Kp2 : Gain  Gain=KP_y
  Kp3 : Gain  Gain=KI_y
  Mux : Mux  Inputs=2
  Scope : Scope
  Scope1 : Scope
  Sum2 : Sum  Inputs=+++
  Sum3 : Sum  Inputs=|-+
  Sum5 : Sum  Inputs=+++
  Sum6 : Sum  Inputs=|-+
  uxy : Outport
  wires:
  X_e (m)/1 -> Sum3/1
  Integrator Limited/1 -> Sum2/1
  Sum2/1 -> Mux/1, Scope/1
  Kp1/1 -> Integrator Limited/1
  Kp/1 -> Sum2/2
  Kp2/1 -> Sum5/2
  Y_e (m)/1 -> Sum6/1
  Integrator Limited1/1 -> Sum5/1
  Sum5/1 -> Mux/2, Scope1/1
  Kp3/1 -> Integrator Limited1/1
  Mux/1 -> uxy/1
  X_d (m)/1 -> Sum3/2
  Discrete Derivative1/1 -> Kd/1
  Sum3/1 -> Discrete Derivative1/1, Kp/1, Kp1/1
  Y_d (m)/1 -> Sum6/2
  Sum6/1 -> Discrete Derivative2/1, Kp2/1, Kp3/1
  Kd1/1 -> Sum5/3
  Discrete Derivative2/1 -> Kd1/1
  Kd/1 -> Sum2/3

== system SIMULINK_FT_SRL_NZS_Tracking_R18b/control system_UAV/Baseline Controller8/Heading controller ==
  yaw_e (rad) : Inport
  yaw_d. (rad) : Inport  Port=2
  Integrator Limited : Integrator  Commented=on  LimitOutput=on  UpperSaturationLimit=0.3  LowerSaturationLimit=-0.3
  Ki : Gain  Commented=on  Gain=0.01
  Sum1 : Sum  Inputs=|-+
  Sum2 : Sum  Inputs=|++
  proportional control gain - yaw : Gain  Gain=0.2
  yaw_rate_d. (rad/s) : Outport
  wires:
  Sum1/1 -> Ki/1, proportional control gain - yaw/1
  yaw_e (rad)/1 -> Sum1/1
  yaw_d. (rad)/1 -> Sum1/2
  proportional control gain - yaw/1 -> Sum2/1
  Integrator Limited/1 -> Sum2/2
  Ki/1 -> Integrator Limited/1
  Sum2/1 -> yaw_rate_d. (rad/s)/1

== system SIMULINK_FT_SRL_NZS_Tracking_R18b/control system_UAV/Baseline Controller8/Height controller  ==
  Z_d. (m) : Inport
  Z_e (m) : Inport  Port=2
  V_z : Inport  Port=3
  Discrete Derivative1 : simulink/Discrete/Discrete Derivative  gainval=1.0  ICPrevScaledInput=0.0  OutMin=[]  OutMax=[]  OutDataType=fixdt(1, 16)  OutScaling=2^-10  DoSatur=off
  Integrator Limited : Integrator  LimitOutput=on  UpperSaturationLimit=0.1  LowerSaturationLimit=-0.1
  Kd : Gain  Gain=kd_z
  Ki : Gain  Gain=ki_z
  Kp : Gain  Gain=kp_z
  Sum2 : Sum  Inputs=+++
  Sum3 : Sum  Inputs=|-+
  Z_velocity_d (m/s) : Outport
  wires:
  Sum3/1 -> Discrete Derivative1/1, Ki/1, Kp/1
  Z_e (m)/1 -> Sum3/1
  Discrete Derivative1/1 -> Kd/1
  Sum2/1 -> Z_velocity_d (m/s)/1
  Kp/1 -> Sum2/2
  Kd/1 -> Sum2/3
  Ki/1 -> Integrator Limited/1
  Integrator Limited/1 -> Sum2/1
  Z_d. (m)/1 -> Sum3/2

== system SIMULINK_FT_SRL_NZS_Tracking_R18b/control system_UAV/Baseline Controller8/Position controller ==
  X_e (m) : Inport
  Y_e (m) : Inport  Port=2
  X_d (m) : Inport  Port=3
  Y_d (m) : Inport  Port=4
  Discrete Derivative1 : simulink/Discrete/Discrete Derivative  gainval=1.0  ICPrevScaledInput=0.0  OutMin=[]  OutMax=[]  OutDataType=fixdt(1, 16)  OutScaling=2^-10  DoSatur=off
  Discrete Derivative2 : simulink/Discrete/Discrete Derivative  gainval=1.0  ICPrevScaledInput=0.0  OutMin=[]  OutMax=[]  OutDataType=fixdt(1, 16)  OutScaling=2^-10  DoSatur=off
  Integrator Limited : Integrator  LimitOutput=on  UpperSaturationLimit=0.5  LowerSaturationLimit=-0.5
  Integrator Limited1 : Integrator  LimitOutput=on  UpperSaturationLimit=0.5  LowerSaturationLimit=-0.5
  Kd : Gain  Gain=KD_x
  Kd1 : Gain  Gain=KD_y
  Kp : Gain  Gain=KP_x
  Kp1 : Gain  Gain=KI_x
  Kp2 : Gain  Gain=KP_y
  Kp3 : Gain  Gain=KI_y
  Mux : Mux  Inputs=2
  Scope : Scope
  Scope1 : Scope
  Sum2 : Sum  Inputs=+++
  Sum3 : Sum  Inputs=|-+
  Sum5 : Sum  Inputs=+++
  Sum6 : Sum  Inputs=|-+
  uxy : Outport
  wires:
  X_e (m)/1 -> Sum3/1
  Integrator Limited/1 -> Sum2/1
  Sum2/1 -> Mux/1, Scope/1
  Kp1/1 -> Integrator Limited/1
  Kp/1 -> Sum2/2
  Kp2/1 -> Sum5/2
  Y_e (m)/1 -> Sum6/1
  Integrator Limited1/1 -> Sum5/1
  Sum5/1 -> Mux/2, Scope1/1
  Kp3/1 -> Integrator Limited1/1
  Mux/1 -> uxy/1
  X_d (m)/1 -> Sum3/2
  Discrete Derivative1/1 -> Kd/1
  Sum3/1 -> Discrete Derivative1/1, Kp/1, Kp1/1
  Y_d (m)/1 -> Sum6/2
  Sum6/1 -> Discrete Derivative2/1, Kp2/1, Kp3/1
  Kd1/1 -> Sum5/3
  Discrete Derivative2/1 -> Kd1/1
  Kd/1 -> Sum2/3

== system SIMULINK_FT_SRL_NZS_Tracking_R18b/control system_UAV/Baseline Controller9/Heading controller ==
  yaw_e (rad) : Inport
  yaw_d. (rad) : Inport  Port=2
  Integrator Limited : Integrator  Commented=on  LimitOutput=on  UpperSaturationLimit=0.3  LowerSaturationLimit=-0.3
  Ki : Gain  Commented=on  Gain=0.01
  Sum1 : Sum  Inputs=|-+
  Sum2 : Sum  Inputs=|++
  proportional control gain - yaw : Gain  Gain=0.2
  yaw_rate_d. (rad/s) : Outport
  wires:
  Sum1/1 -> Ki/1, proportional control gain - yaw/1
  yaw_e (rad)/1 -> Sum1/1
  yaw_d. (rad)/1 -> Sum1/2
  proportional control gain - yaw/1 -> Sum2/1
  Integrator Limited/1 -> Sum2/2
  Ki/1 -> Integrator Limited/1
  Sum2/1 -> yaw_rate_d. (rad/s)/1

== system SIMULINK_FT_SRL_NZS_Tracking_R18b/control system_UAV/Baseline Controller9/Height controller  ==
  Z_d. (m) : Inport
  Z_e (m) : Inport  Port=2
  V_z : Inport  Port=3
  Discrete Derivative1 : simulink/Discrete/Discrete Derivative  gainval=1.0  ICPrevScaledInput=0.0  OutMin=[]  OutMax=[]  OutDataType=fixdt(1, 16)  OutScaling=2^-10  DoSatur=off
  Integrator Limited : Integrator  LimitOutput=on  UpperSaturationLimit=0.1  LowerSaturationLimit=-0.1
  Kd : Gain  Gain=kd_z
  Ki : Gain  Gain=ki_z
  Kp : Gain  Gain=kp_z
  Sum2 : Sum  Inputs=+++
  Sum3 : Sum  Inputs=|-+
  Z_velocity_d (m/s) : Outport
  wires:
  Sum3/1 -> Discrete Derivative1/1, Ki/1, Kp/1
  Z_e (m)/1 -> Sum3/1
  Discrete Derivative1/1 -> Kd/1
  Sum2/1 -> Z_velocity_d (m/s)/1
  Kp/1 -> Sum2/2
  Kd/1 -> Sum2/3
  Ki/1 -> Integrator Limited/1
  Integrator Limited/1 -> Sum2/1
  Z_d. (m)/1 -> Sum3/2

== system SIMULINK_FT_SRL_NZS_Tracking_R18b/control system_UAV/Baseline Controller9/Position controller ==
  X_e (m) : Inport
  Y_e (m) : Inport  Port=2
  X_d (m) : Inport  Port=3
  Y_d (m) : Inport  Port=4
  Discrete Derivative1 : simulink/Discrete/Discrete Derivative  gainval=1.0  ICPrevScaledInput=0.0  OutMin=[]  OutMax=[]  OutDataType=fixdt(1, 16)  OutScaling=2^-10  DoSatur=off
  Discrete Derivative2 : simulink/Discrete/Discrete Derivative  gainval=1.0  ICPrevScaledInput=0.0  OutMin=[]  OutMax=[]  OutDataType=fixdt(1, 16)  OutScaling=2^-10  DoSatur=off
  Integrator Limited : Integrator  LimitOutput=on  UpperSaturationLimit=0.5  LowerSaturationLimit=-0.5
  Integrator Limited1 : Integrator  LimitOutput=on  UpperSaturationLimit=0.5  LowerSaturationLimit=-0.5
  Kd : Gain  Gain=KD_x
  Kd1 : Gain  Gain=KD_y
  Kp : Gain  Gain=KP_x
  Kp1 : Gain  Gain=KI_x
  Kp2 : Gain  Gain=KP_y
  Kp3 : Gain  Gain=KI_y
  Mux : Mux  Inputs=2
  Scope : Scope
  Scope1 : Scope
  Sum2 : Sum  Inputs=+++
  Sum3 : Sum  Inputs=|-+
  Sum5 : Sum  Inputs=+++
  Sum6 : Sum  Inputs=|-+
  uxy : Outport
  wires:
  X_e (m)/1 -> Sum3/1
  Integrator Limited/1 -> Sum2/1
  Sum2/1 -> Mux/1, Scope/1
  Kp1/1 -> Integrator Limited/1
  Kp/1 -> Sum2/2
  Kp2/1 -> Sum5/2
  Y_e (m)/1 -> Sum6/1
  Integrator Limited1/1 -> Sum5/1
  Sum5/1 -> Mux/2, Scope1/1
  Kp3/1 -> Integrator Limited1/1
  Mux/1 -> uxy/1
  X_d (m)/1 -> Sum3/2
  Discrete Derivative1/1 -> Kd/1
  Sum3/1 -> Discrete Derivative1/1, Kp/1, Kp1/1
  Y_d (m)/1 -> Sum6/2
  Sum6/1 -> Discrete Derivative2/1, Kp2/1, Kp3/1
  Kd1/1 -> Sum5/3
  Discrete Derivative2/1 -> Kd1/1
  Kd/1 -> Sum2/3

== system SIMULINK_FT_SRL_NZS_Tracking_R18b/control system_car1/Baseline Controller1/Heading controller ==
  yaw_e (rad) : Inport
  yaw_d. (rad) : Inport  Port=2
  Integrator Limited : Integrator  Commented=on  LimitOutput=on  UpperSaturationLimit=0.3  LowerSaturationLimit=-0.3
  Ki : Gain  Commented=on  Gain=0.01
  Sum1 : Sum  Inputs=|-+
  Sum2 : Sum  Inputs=|++
  proportional control gain - yaw : Gain  Gain=0.2
  yaw_rate_d. (rad/s) : Outport
  wires:
  Sum1/1 -> Ki/1, proportional control gain - yaw/1
  yaw_e (rad)/1 -> Sum1/1
  yaw_d. (rad)/1 -> Sum1/2
  proportional control gain - yaw/1 -> Sum2/1
  Integrator Limited/1 -> Sum2/2
  Ki/1 -> Integrator Limited/1
  Sum2/1 -> yaw_rate_d. (rad/s)/1

== system SIMULINK_FT_SRL_NZS_Tracking_R18b/control system_car1/Baseline Controller1/Height controller  ==
  Z_d. (m) : Inport
  Z_e (m) : Inport  Port=2
  V_z : Inport  Port=3
  Discrete Derivative1 : simulink/Discrete/Discrete Derivative  gainval=1.0  ICPrevScaledInput=0.0  OutMin=[]  OutMax=[]  OutDataType=fixdt(1, 16)  OutScaling=2^-10  DoSatur=off
  Integrator Limited : Integrator  LimitOutput=on  UpperSaturationLimit=0.1  LowerSaturationLimit=-0.1
  Kd : Gain  Gain=kd_z
  Ki : Gain  Gain=ki_z
  Kp : Gain  Gain=kp_z
  Sum2 : Sum  Inputs=+++
  Sum3 : Sum  Inputs=|-+
  Z_velocity_d (m/s) : Outport
  wires:
  Sum3/1 -> Discrete Derivative1/1, Ki/1, Kp/1
  Z_e (m)/1 -> Sum3/1
  Discrete Derivative1/1 -> Kd/1
  Sum2/1 -> Z_velocity_d (m/s)/1
  Kp/1 -> Sum2/2
  Kd/1 -> Sum2/3
  Ki/1 -> Integrator Limited/1
  Integrator Limited/1 -> Sum2/1
  Z_d. (m)/1 -> Sum3/2
